simulink model "gm_sampleModel1427_4_sub_sub_sub"  (R2023a)
settings: Solver=VariableStepAuto  StartTime=0.0  StopTime=10.0  RelTol=1e-3
libraries: hdlsllib x6, simulink x3
settings Model: Creator=user1  LastModifiedBy=user1
settings OptimizationCC: BlockReduction=off  ConditionallyExecuteInputs=off
settings DebuggingCC: InheritedTsInSrcMsg=none

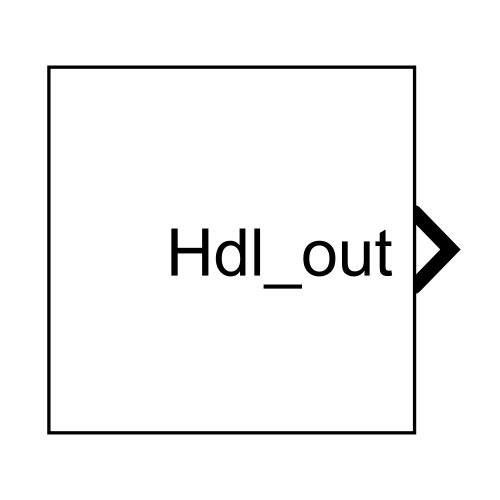
[thumbnail: Simulink's stored preview of the top-level diagram]
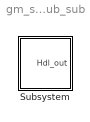
== system gm_sampleModel1427_4_sub_sub_sub ==
  Subsystem : Subsystem

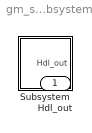
== system gm_sampleModel1427_4_sub_sub_sub/Subsystem ==
  Subsystem : Subsystem
  Hdl_out : Outport  OutDataTypeStr=uint8

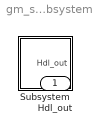
== system gm_sampleModel1427_4_sub_sub_sub/Subsystem/Subsystem ==
  Subsystem : Subsystem
  Hdl_out : Outport  OutDataTypeStr=uint8

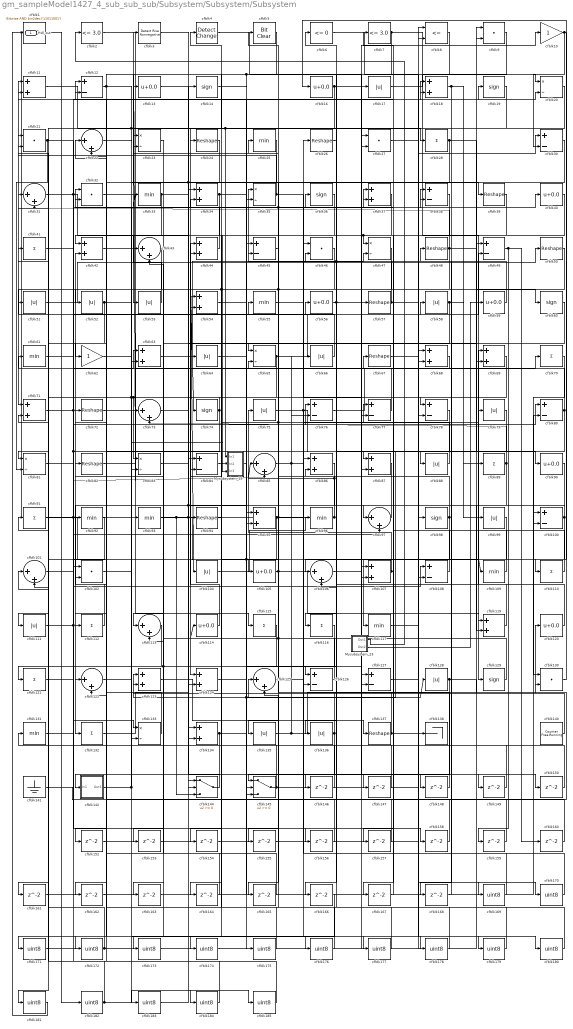
== system gm_sampleModel1427_4_sub_sub_sub/Subsystem/Subsystem/Subsystem ==
  Mysubsystem_19 : Subsystem  TreatAsAtomicUnit=on  RTWFcnName=Mysubsystem_19
      settings: RTWFcnNameOpts=User specified  RTWFileNameOpts=Use function name
  Mysubsystem_23 : Subsystem  TreatAsAtomicUnit=on  RTWFcnName=Mysubsystem_23
      settings: RTWFcnNameOpts=User specified  RTWFileNameOpts=Use function name
  cfblk1 : simulink/Logic and Bit Operations/Bitwise Operator  logicop=AND  UseBitMask=on  BitMask=bin2dec('11011001')  BitMaskRealWorld=Stored Integer
      settings: LibrarySourceBlock=|
      | hdlsllib/Logic and Bit
      | Operations/Bitwise
      | Operator
  cfblk10 : Gain  OutDataTypeStr=uint8
  cfblk{12,30,38,45,49,76..78,80,84,100,108,126..127} (14 alike) : Sum  Inputs=+-  OutDataTypeStr=uint8
  cfblk{22,31,43,73,85,97,101,106,113,122,125} (11 alike) : Sum  Inputs=|++  OutDataTypeStr=uint8
  cfblk{9,21,27,32,46,102,130} (7 alike) : DotProduct  OutDataTypeStr=uint8
  cfblk{17,51..53,58,64,66,75,79,88,99,104,111,128,135..136} (16 alike) : Abs  OutDataTypeStr=uint8  SaturateOnIntegerOverflow=off
  cfblk{13,16,40,56,59,90,105,114,120} (9 alike) : Bias  Bias=0.0  SaturateOnIntegerOverflow=off
  cfblk{11,18,34,37,42,44,54,63,68..69,71,86..87,95,107,119,123..124,134} (19 alike) : Sum  OutDataTypeStr=uint8
  cfblk{25,33,55,61,92..93,96,109,117,131} (10 alike) : MinMax  OutDataTypeStr=uint8
  cfblk{28,41,70,89,91,110,112,115..116,121,132} (11 alike) : Sum  Inputs=+  OutDataTypeStr=uint8
  cfblk{14,19,36,60,74,98,129} (7 alike) : Signum
  cfblk{20,23,35,47,65,81,83,133} (8 alike) : Product  Inputs=*/  OutDataTypeStr=uint8  RndMeth=Zero  SaturateOnIntegerOverflow=on
  cfblk{24,26,39,48,50,57,67,72,82,94,137} (11 alike) : Reshape
  cfblk138 : Terminator
  cfblk140 : hdlsllib/Sources/Counter Free-Running  NumBits=16  tsamp=-1
  cfblk141 : Ground
  cfblk142 : Subsystem
      settings: LibrarySourceBlock=|
      | hdlsllib/Ports &
      | Subsystems/Subsystem
  cfblk144 : Switch  OutDataTypeStr=uint8  SaturateOnIntegerOverflow=off  InputSameDT=off
  cfblk145 : Switch  OutDataTypeStr=uint8  SaturateOnIntegerOverflow=off  InputSameDT=off
  cfblk{146..150,152..168} (22 alike) : Delay  SampleTime=1
  cfblk{169..185} (17 alike) : DataTypeConversion  OutDataTypeStr=uint8  SaturateOnIntegerOverflow=off  RndMeth=Floor
  cfblk2 : hdlsllib/Logic and Bit Operations/Compare To Constant  relop=<=  const=3.0  OutDataTypeStr=uint8
  cfblk3 : hdlsllib/Logic and Bit Operations/Detect Rise Nonnegative  vinit=0  OutDataTypeStr=uint8
  cfblk4 : simulink/Logic and Bit Operations/Detect Change  vinit=0  OutDataTypeStr=uint8
      settings: LibrarySourceBlock=|
      | hdlsllib/Logic and Bit
      | Operations/Detect
      | Change
  cfblk5 : simulink/Logic and Bit Operations/Bit Clear  iBit=0
      settings: LibrarySourceBlock=|
      | hdlsllib/Logic and Bit
      | Operations/Bit Clear
  cfblk6 : hdlsllib/Logic and Bit Operations/Compare To Zero  relop=<=  OutDataTypeStr=uint8
  cfblk62 : Gain  OutDataTypeStr=uint8
  cfblk7 : hdlsllib/Logic and Bit Operations/Compare To Constant  relop=<=  const=3.0  OutDataTypeStr=uint8
  cfblk8 : RelationalOperator  Operator=<=  OutDataTypeStr=boolean  InputSameDT=off
  Hdl_out : Outport  OutDataTypeStr=uint8
  wires:
  Mysubsystem_23/2(Out2) -> cfblk59/1
  Mysubsystem_23/1(Out1) -> cfblk2/1
  cfblk36/1 -> Mysubsystem_19/2(In2)
  cfblk185/1 -> cfblk102/2
  cfblk162/1 -> cfblk185/1
  cfblk184/1 -> cfblk102/1
  cfblk183/1 -> cfblk144/1
  cfblk102/1 -> cfblk183/1
  cfblk182/1 -> cfblk91/1, cfblk184/1
  cfblk181/1 -> cfblk1/1
  cfblk166/1 -> cfblk181/1
  cfblk180/1 -> cfblk125/2
  cfblk22/1 -> cfblk180/1
  cfblk179/1 -> cfblk125/1
  cfblk178/1 -> cfblk46/2
  cfblk125/1 -> cfblk178/1
  cfblk177/1 -> cfblk84/2
  cfblk176/1 -> cfblk84/1
  cfblk154/1 -> cfblk176/1
  cfblk175/1 -> cfblk72/1
  cfblk84/1 -> cfblk175/1
  cfblk174/1 -> cfblk9/2
  cfblk90/1 -> cfblk174/1
  cfblk173/1 -> cfblk9/1
  cfblk172/1 -> cfblk131/1, cfblk68/2
  cfblk171/1 -> cfblk27/2
  cfblk113/1 -> cfblk171/1
  cfblk170/1 -> cfblk27/1
  cfblk117/1 -> cfblk170/1
  cfblk169/1 -> cfblk46/1
  cfblk27/1 -> cfblk169/1
  cfblk168/1 -> cfblk48/1
  cfblk60/1 -> cfblk168/1
  cfblk167/1 -> cfblk7/1
  cfblk79/1 -> cfblk167/1
  cfblk165/1 -> cfblk122/2
  cfblk164/1 -> cfblk43/2
  cfblk163/1 -> cfblk145/2
  cfblk161/1 -> cfblk80/2
  cfblk160/1 -> cfblk12/2
  cfblk159/1 -> cfblk45/1
  cfblk158/1 -> cfblk54/2
  cfblk157/1 -> cfblk144/2
  cfblk99/1 -> cfblk157/1
  cfblk156/1 -> cfblk34/1
  cfblk155/1 -> cfblk8/2
  cfblk153/1 -> cfblk124/2
  cfblk23/1 -> cfblk153/1
  cfblk152/1 -> cfblk127/1
  cfblk150/1 -> cfblk71/2
  cfblk3/1 -> cfblk150/1
  cfblk149/1 -> cfblk107/1
  cfblk148/1 -> cfblk86/1
  cfblk147/1 -> cfblk22/1
  cfblk38/1 -> cfblk147/1
  cfblk146/1 -> cfblk101/1
  cfblk78/1 -> cfblk146/1
  cfblk136/1 -> cfblk13/1, cfblk33/1, cfblk155/1
  cfblk71/1 -> cfblk38/1, cfblk107/2
  cfblk59/1 -> cfblk5/1, cfblk36/1
  cfblk70/1 -> cfblk100/2
  cfblk128/1 -> cfblk130/2, cfblk166/1
  cfblk43/1 -> cfblk92/1
  cfblk89/1 -> cfblk119/2, cfblk73/2
  cfblk10/1 -> cfblk110/1, cfblk30/2
  cfblk8/1 -> cfblk24/1
  cfblk133/1 -> cfblk51/1
  cfblk28/1 -> cfblk52/1, cfblk90/1
  cfblk44/1 -> cfblk23/2
  cfblk115/1 -> cfblk133/2
  cfblk131/1 -> cfblk76/1
  cfblk142/1(Out1) -> cfblk38/2, cfblk177/1
  cfblk40/1 -> cfblk105/1
  cfblk94/1 -> cfblk4/1
  cfblk4/1 -> cfblk57/1
  cfblk101/1 -> cfblk19/1
  cfblk67/1 -> cfblk30/1
  cfblk14/1 -> cfblk127/2, cfblk109/1
  cfblk83/1 -> cfblk20/2
  cfblk25/1 -> cfblk35/2
  cfblk105/1 -> cfblk119/1, cfblk165/1
  cfblk96/1 -> cfblk11/2, cfblk85/1, Hdl_out/1
  cfblk26/1 -> cfblk136/1
  cfblk135/1 -> cfblk100/1, cfblk66/1
  cfblk49/1 -> cfblk159/1, cfblk160/1
  cfblk65/1 -> Mysubsystem_19/3(In3), cfblk121/1, cfblk49/2
  cfblk21/1 -> cfblk133/1, cfblk81/2
  cfblk121/1 -> cfblk108/1
  cfblk92/1 -> cfblk101/2
  cfblk91/1 -> cfblk117/1, cfblk108/2, cfblk63/1
  cfblk24/1 -> cfblk122/1, cfblk134/2
  cfblk20/1 -> Mysubsystem_19/1(In1), cfblk22/2, cfblk63/2
  cfblk98/1 -> cfblk23/1, cfblk116/1
  cfblk16/1 -> cfblk81/1, cfblk149/1
  cfblk64/1 -> cfblk47/2
  cfblk74/1 -> cfblk112/1, cfblk73/1
  cfblk73/1 -> cfblk94/1, cfblk95/2
  cfblk62/1 -> cfblk43/1
  cfblk72/1 -> cfblk87/2
  cfblk81/1 -> cfblk97/2
  cfblk55/1 -> cfblk26/1
  cfblk61/1 -> cfblk83/2, cfblk85/2
  cfblk51/1 -> cfblk50/1
  cfblk120/1 -> cfblk32/2
  cfblk87/1 -> cfblk86/2
  cfblk6/1 -> cfblk78/2
  cfblk52/1 -> cfblk111/1, cfblk158/1
  cfblk45/1 -> cfblk145/1
  cfblk68/1 -> cfblk65/2
  cfblk35/1 -> cfblk21/2, cfblk77/2
  cfblk41/1 -> cfblk88/1
  cfblk129/1 -> cfblk61/1
  cfblk126/1 -> cfblk82/1
  cfblk77/1 -> cfblk21/1
  cfblk116/1 -> cfblk162/1, cfblk163/1
  cfblk108/1 -> cfblk32/1
  cfblk1/1 -> cfblk182/1
  cfblk31/1 -> cfblk134/1, cfblk37/2
  cfblk37/1 -> cfblk53/1
  cfblk30/1 -> cfblk65/1
  cfblk85/1 -> cfblk79/1, cfblk76/2
  cfblk106/1 -> cfblk17/1
  cfblk69/1 -> cfblk83/1, cfblk161/1
  cfblk9/1 -> cfblk172/1
  cfblk137/1 -> cfblk34/2, cfblk114/1, cfblk40/1
  cfblk11/1 -> cfblk68/1
  cfblk122/1 -> cfblk80/1
  cfblk141/1 -> cfblk120/1
  cfblk82/1 -> cfblk70/1
  cfblk18/1 -> cfblk78/1, cfblk89/1
  cfblk124/1 -> cfblk56/1
  cfblk63/1 -> cfblk35/1
  cfblk145/1 -> cfblk41/1, cfblk98/1
  cfblk50/1 -> cfblk113/2
  cfblk53/1 -> cfblk3/1
  cfblk140/1 -> cfblk123/2
  cfblk100/1 -> cfblk97/1, cfblk106/1
  cfblk110/1 -> cfblk12/1
  cfblk86/1 -> cfblk132/1
  cfblk76/1 -> cfblk49/1
  cfblk17/1 -> cfblk20/1
  cfblk5/1 -> cfblk93/1, cfblk145/3
  cfblk95/1 -> cfblk77/1, cfblk55/1, cfblk154/1
  cfblk119/1 -> cfblk69/1
  cfblk134/1 -> cfblk18/2, cfblk128/1, cfblk173/1
  cfblk58/1 -> cfblk113/1, cfblk99/1
  cfblk13/1 -> cfblk28/1
  cfblk75/1 -> cfblk130/1, cfblk148/1
  cfblk54/1 -> cfblk95/1
  cfblk46/1 -> cfblk71/1
  cfblk42/1 -> cfblk44/2
  cfblk7/1 -> cfblk129/1, cfblk106/2
  cfblk47/1 -> cfblk74/1, cfblk164/1
  cfblk93/1 -> cfblk138/1, cfblk18/1, cfblk144/3
  cfblk132/1 -> cfblk14/1
  cfblk130/1 -> cfblk16/1
  cfblk2/1 -> cfblk87/1
  cfblk97/1 -> cfblk6/1
  cfblk32/1 -> cfblk115/1
  cfblk66/1 -> cfblk11/1
  cfblk34/1 -> cfblk62/1, cfblk126/2
  cfblk48/1 -> cfblk104/1, cfblk135/1, cfblk31/2, cfblk60/1
  cfblk109/1 -> cfblk67/1
  cfblk112/1 -> cfblk42/2
  cfblk114/1 -> cfblk44/1
  cfblk111/1 -> cfblk58/1, cfblk156/1
  cfblk127/1 -> cfblk8/1
  cfblk88/1 -> cfblk25/1, cfblk54/1
  cfblk39/1 -> cfblk47/1, cfblk64/1
  cfblk19/1 -> cfblk124/1
  cfblk123/1 -> cfblk137/1
  cfblk80/1 -> cfblk123/1, cfblk31/1
  cfblk56/1 -> cfblk126/1, cfblk10/1
  cfblk104/1 -> cfblk96/1
  cfblk57/1 -> cfblk45/2, cfblk179/1
  cfblk33/1 -> cfblk42/1, cfblk69/2
  cfblk107/1 -> cfblk75/1, cfblk37/1
  cfblk144/1 -> cfblk142/1(In1)
  cfblk12/1 -> cfblk39/1, cfblk152/1

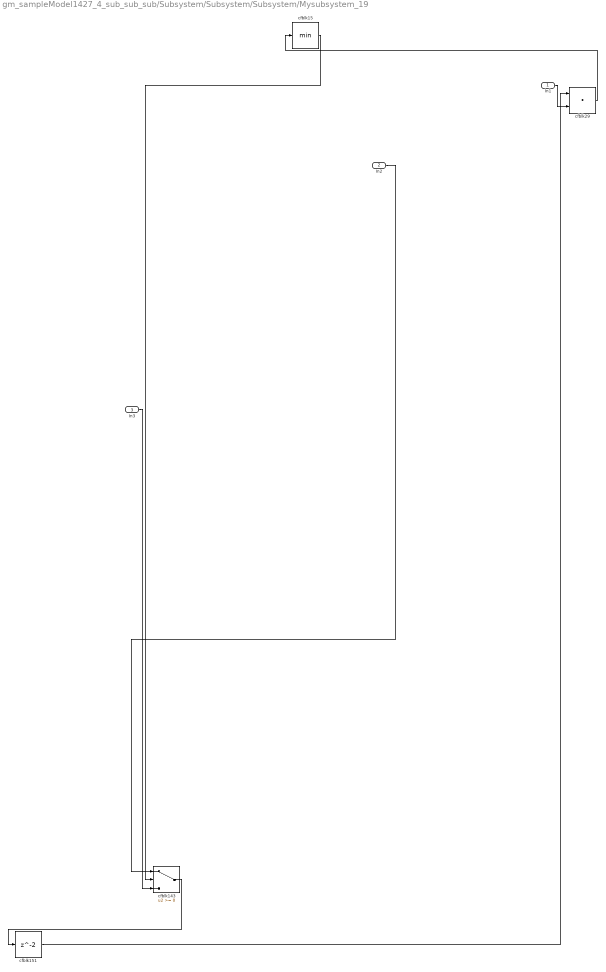
== system gm_sampleModel1427_4_sub_sub_sub/Subsystem/Subsystem/Subsystem/Mysubsystem_19 ==
  In1 : Inport
  In2 : Inport  Port=2
  In3 : Inport  Port=3
  cfblk143 : Switch  SaturateOnIntegerOverflow=off  InputSameDT=off
  cfblk15 : MinMax
  cfblk151 : Delay  SampleTime=1
  cfblk29 : DotProduct  OutDataTypeStr=Inherit: Inherit via internal rule
  wires:
  cfblk151/1 -> cfblk29/1
  cfblk143/1 -> cfblk151/1
  cfblk15/1 -> cfblk143/2
  cfblk29/1 -> cfblk15/1
  In3/1 -> cfblk143/3
  In1/1 -> cfblk29/2
  In2/1 -> cfblk143/1

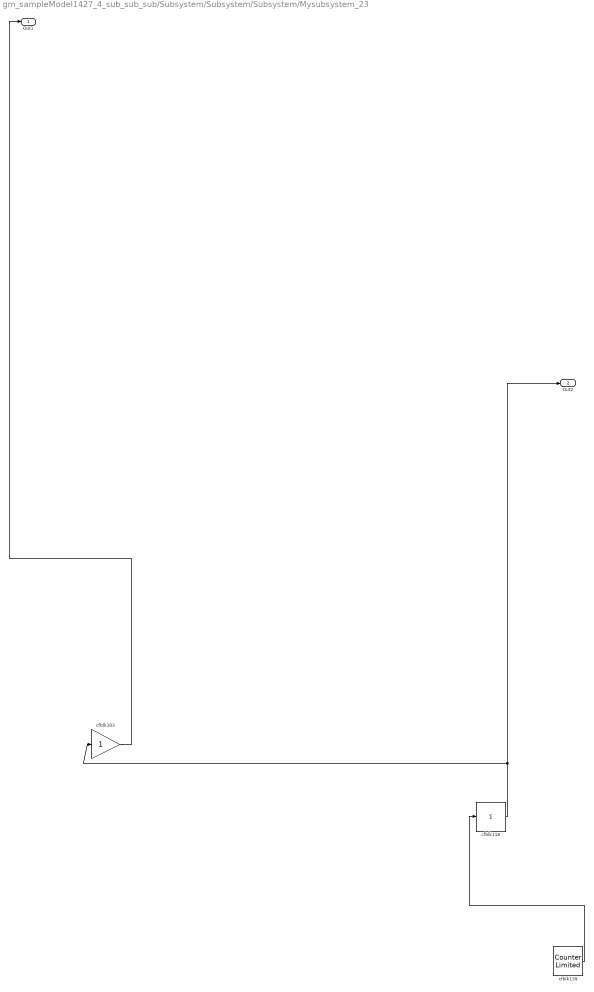
== system gm_sampleModel1427_4_sub_sub_sub/Subsystem/Subsystem/Subsystem/Mysubsystem_23 ==
  cfblk103 : Gain
  cfblk118 : Sum  Inputs=+
  cfblk139 : hdlsllib/Sources/Counter Limited  uplimit=7  tsamp=-1
  Out1 : Outport
  Out2 : Outport  Port=2
  wires:
  cfblk118/1 -> Out2/1, cfblk103/1
  cfblk139/1 -> cfblk118/1
  cfblk103/1 -> Out1/1

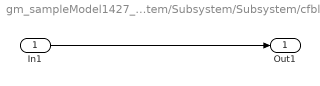
== system gm_sampleModel1427_4_sub_sub_sub/Subsystem/Subsystem/Subsystem/cfblk142 ==
  In1 : Inport
  Out1 : Outport
  wires:
  In1/1 -> Out1/1
